simulink model "lab3"  (R2022b)
settings: Solver=VariableStepAuto  StartTime=0.0  StopTime=10.0  RelTol=1e-3
values from neighbouring files (symbols this model uses):
  Beq = 1.9610e-06    (= 1.961e-06)    [parameters.m]
  deg2V = 2.5/170    (= 0.0147058823529)    [parameters.m]
  Jeq = 8.4138e-07    [parameters.m]
  rads2rpm = 60/2/pi    (= 9.54929658551)    [parameters.m]
  V2deg = 170/2.5    (= 68)    [parameters.m]
undefined symbols (not defined in the file or in its folder): drv, gbox, mld, mot, sens
settings Model: Creator=gugli  LastModifiedBy=gugli

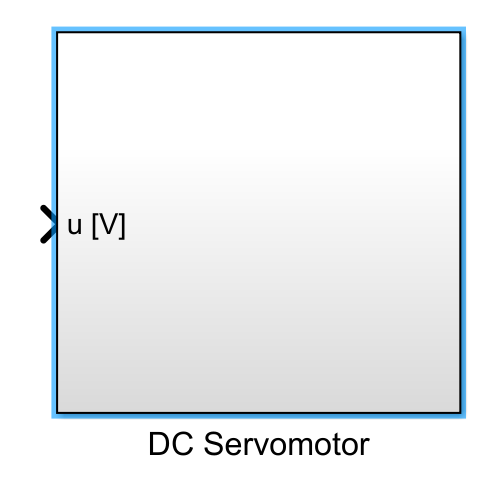
[thumbnail: Simulink's stored preview of the top-level diagram]
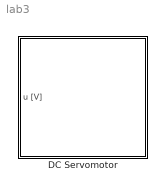
== system lab3 ==
  DC Servomotor : Subsystem

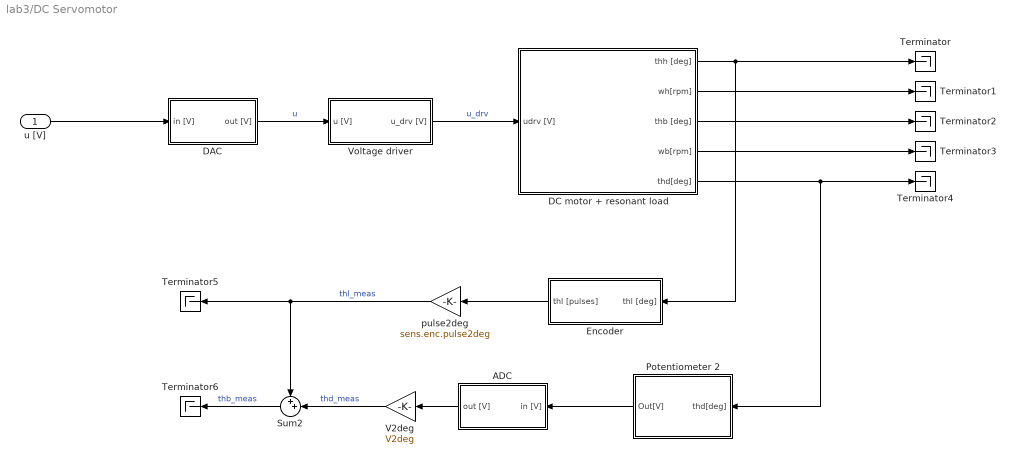
== system lab3/DC Servomotor ==
  u [V] : Inport
  ADC : Subsystem
  DAC : Subsystem
  DC motor + resonant load : Subsystem
  Encoder : Subsystem
  Potentiometer 2 : Subsystem
  Sum2 : Sum  Inputs=++|
  Terminator{,1..6} (7 alike) : Terminator
  V2deg : Gain  Gain=V2deg
  Voltage driver : Subsystem
  pulse2deg : Gain  Gain=sens.enc.pulse2deg
  wires:
  Encoder/1(thl [pulses]) -> pulse2deg/1
  DAC/1(out [V]) -> Voltage driver/1(u [V])  "u"
  pulse2deg/1 -> Sum2/1, Terminator5/1  "thl_meas"
  u [V]/1 -> DAC/1(in [V])
  DC motor + resonant load/1(thh [deg]) -> Encoder/1(thl [deg]), Terminator/1
  DC motor + resonant load/2(wh[rpm]) -> Terminator1/1
  Voltage driver/1(u_drv [V]) -> DC motor + resonant load/1(udrv [V])  "u_drv"
  DC motor + resonant load/3(thb [deg]) -> Terminator2/1
  DC motor + resonant load/4(wb[rpm]) -> Terminator3/1
  DC motor + resonant load/5(thd[deg]) -> Potentiometer 2/1(thd[deg]), Terminator4/1
  Potentiometer 2/1(Out[V]) -> ADC/1(in [V])
  ADC/1(out [V]) -> V2deg/1
  V2deg/1 -> Sum2/2  "thd_meas"
  Sum2/1 -> Terminator6/1  "thb_meas"

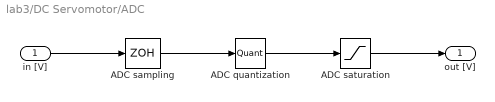
== system lab3/DC Servomotor/ADC ==
  in [V] : Inport
  ADC quantization : Quantizer  QuantizationInterval=daq.adc.q
  ADC sampling : ZeroOrderHold  SampleTime=0.001
  ADC saturation : Saturate  UpperLimit=10  LowerLimit=-10
  out [V] : Outport
  wires:
  ADC saturation/1 -> out [V]/1
  ADC quantization/1 -> ADC saturation/1
  in [V]/1 -> ADC sampling/1
  ADC sampling/1 -> ADC quantization/1

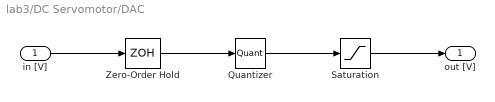
== system lab3/DC Servomotor/DAC ==
  in [V] : Inport
  Quantizer : Quantizer  QuantizationInterval=daq.dac.q
  Saturation : Saturate  UpperLimit=10  LowerLimit=-10
  Zero-Order Hold : ZeroOrderHold  SampleTime=0.001
  out [V] : Outport
  wires:
  Saturation/1 -> out [V]/1
  Quantizer/1 -> Saturation/1
  in [V]/1 -> Zero-Order Hold/1
  Zero-Order Hold/1 -> Quantizer/1

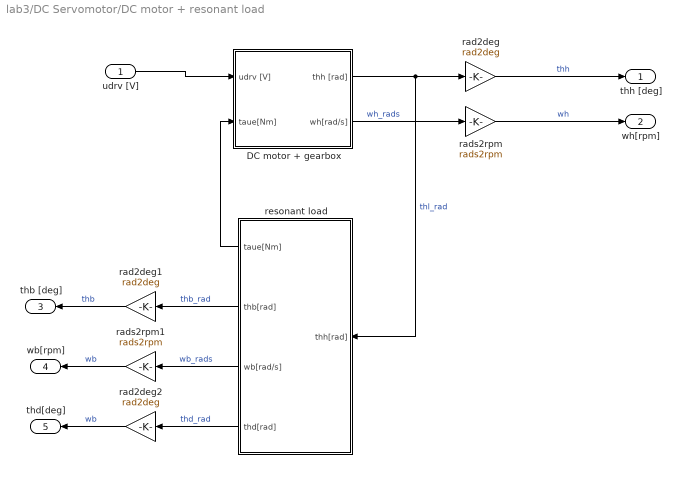
== system lab3/DC Servomotor/DC motor + resonant load ==
  udrv [V] : Inport
  DC motor + gearbox : Subsystem
  rad2deg : Gain  Gain=rad2deg
  rad2deg1 : Gain  Gain=rad2deg
  rad2deg2 : Gain  Gain=rad2deg
  rads2rpm : Gain  Gain=rads2rpm
  rads2rpm1 : Gain  Gain=rads2rpm
  resonant load : Subsystem
  thh [deg] : Outport
  wh[rpm] : Outport  Port=2
  thb [deg] : Outport  Port=3
  wb[rpm] : Outport  Port=4
  thd[deg] : Outport  Port=5
  wires:
  DC motor + gearbox/1(thh [rad]) -> resonant load/1(thh[rad]), rad2deg/1  "thl_rad"
  rad2deg2/1 -> thd[deg]/1  "wb"
  resonant load/1(taue[Nm]) -> DC motor + gearbox/2(taue[Nm])
  DC motor + gearbox/2(wh[rad/s]) -> rads2rpm/1  "wh_rads"
  rad2deg/1 -> thh [deg]/1  "thh"
  resonant load/4(thd[rad]) -> rad2deg2/1  "thd_rad"
  rads2rpm/1 -> wh[rpm]/1  "wh"
  udrv [V]/1 -> DC motor + gearbox/1(udrv [V])
  resonant load/2(thb[rad]) -> rad2deg1/1  "thb_rad"
  resonant load/3(wb[rad/s]) -> rads2rpm1/1  "wb_rads"
  rads2rpm1/1 -> wb[rpm]/1  "wb"
  rad2deg1/1 -> thb [deg]/1  "thb"

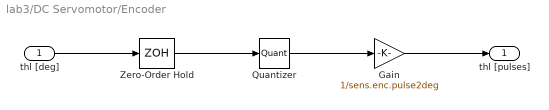
== system lab3/DC Servomotor/Encoder ==
  thl [deg] : Inport
  Gain : Gain  Gain=1/sens.enc.pulse2deg
  Quantizer : Quantizer  QuantizationInterval=sens.enc.pulse2deg
  Zero-Order Hold : ZeroOrderHold  SampleTime=0.001
  thl [pulses] : Outport
  wires:
  Zero-Order Hold/1 -> Quantizer/1
  thl [deg]/1 -> Zero-Order Hold/1
  Quantizer/1 -> Gain/1
  Gain/1 -> thl [pulses]/1

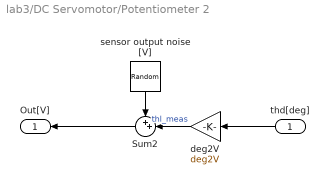
== system lab3/DC Servomotor/Potentiometer 2 ==
  thd[deg] : Inport
  Sum2 : Sum  Inputs=++|
  deg2V : Gain  Gain=deg2V
  sensor output noise [V] : RandomNumber  Variance=3.5*10^[-7]  SampleTime=0.001
  Out[V] : Outport
  wires:
  Sum2/1 -> Out[V]/1
  sensor output noise [V]/1 -> Sum2/1
  deg2V/1 -> Sum2/2  "thl_meas"
  thd[deg]/1 -> deg2V/1

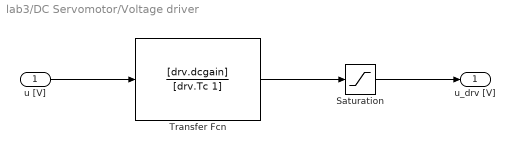
== system lab3/DC Servomotor/Voltage driver ==
  u [V] : Inport
  Saturation : Saturate  UpperLimit=12  LowerLimit=-12
  Transfer Fcn : TransferFcn  Numerator=[drv.dcgain]  Denominator=[drv.Tc 1]
  u_drv [V] : Outport
  wires:
  Saturation/1 -> u_drv [V]/1
  Transfer Fcn/1 -> Saturation/1
  u [V]/1 -> Transfer Fcn/1

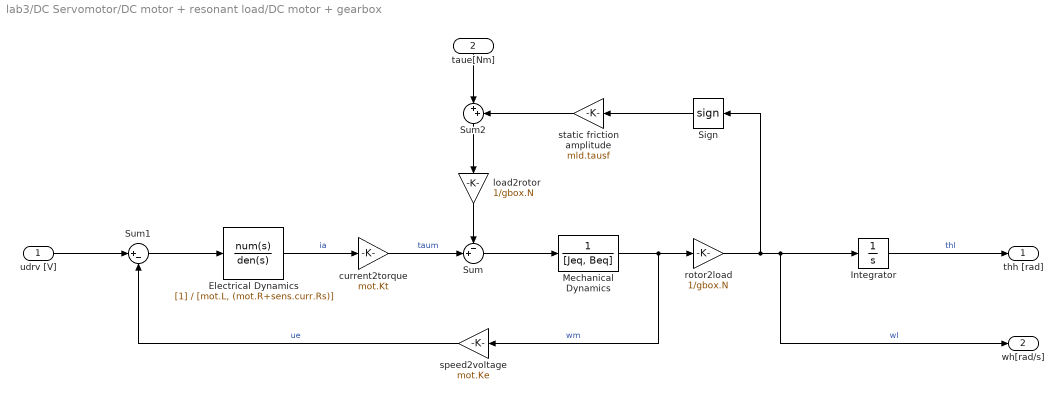
== system lab3/DC Servomotor/DC motor + resonant load/DC motor + gearbox ==
  udrv [V] : Inport
  taue[Nm] : Inport  Port=2
  Electrical Dynamics : TransferFcn  Denominator=[mot.L, (mot.R+sens.curr.Rs)]
  Integrator : Integrator
  Mechanical Dynamics : TransferFcn  Denominator=[Jeq, Beq]
  Sign : Signum  ZeroCross=off
  Sum : Sum  Inputs=-+|
  Sum1 : Sum  Inputs=|+-
  Sum2 : Sum  Inputs=|++
  current2torque : Gain  Gain=mot.Kt
  load2rotor : Gain  Gain=1/gbox.N
  rotor2load : Gain  Gain=1/gbox.N
  speed2voltage : Gain  Gain=mot.Ke
  static friction amplitude : Gain  Gain=mld.tausf
  thh [rad] : Outport
  wh[rad/s] : Outport  Port=2
  wires:
  udrv [V]/1 -> Sum1/1
  load2rotor/1 -> Sum/1
  Sign/1 -> static friction amplitude/1
  Electrical Dynamics/1 -> current2torque/1  "ia"
  current2torque/1 -> Sum/2  "taum"
  speed2voltage/1 -> Sum1/2  "ue"
  Mechanical Dynamics/1 -> rotor2load/1, speed2voltage/1  "wm"
  Integrator/1 -> thh [rad]/1  "thl"
  Sum1/1 -> Electrical Dynamics/1
  rotor2load/1 -> wh[rad/s]/1, Integrator/1, Sign/1  "wl"
  Sum/1 -> Mechanical Dynamics/1
  static friction amplitude/1 -> Sum2/2
  Sum2/1 -> load2rotor/1
  taue[Nm]/1 -> Sum2/1

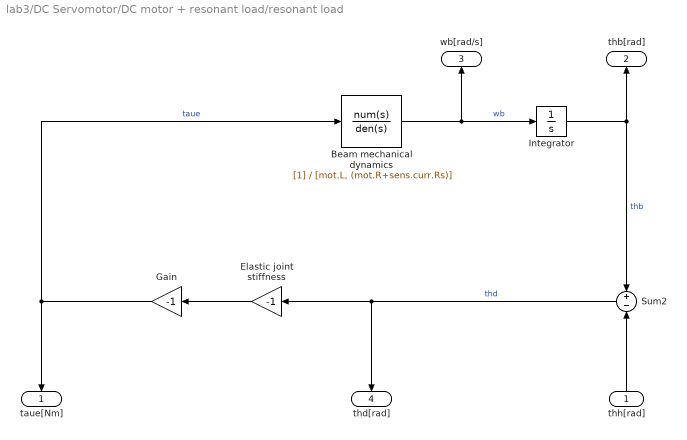
== system lab3/DC Servomotor/DC motor + resonant load/resonant load ==
  thh[rad] : Inport
  Beam mechanical dynamics : TransferFcn  Denominator=[mot.L, (mot.R+sens.curr.Rs)]
  Elastic joint stiffness : Gain  Gain=-1
  Gain : Gain  Gain=-1
  Integrator : Integrator
  Sum2 : Sum  Inputs=+-
  taue[Nm] : Outport
  thb[rad] : Outport  Port=2
  wb[rad/s] : Outport  Port=3
  thd[rad] : Outport  Port=4
  wires:
  Gain/1 -> taue[Nm]/1, Beam mechanical dynamics/1  "taue"
  Elastic joint stiffness/1 -> Gain/1
  Sum2/1 -> thd[rad]/1, Elastic joint stiffness/1  "thd"
  thh[rad]/1 -> Sum2/2
  Integrator/1 -> Sum2/1, thb[rad]/1  "thb"
  Beam mechanical dynamics/1 -> wb[rad/s]/1, Integrator/1  "wb"
